simulink model "slave_ctrl"  (Simulink 6.4)
settings: Solver=FixedStepDiscrete  SolverMode=SingleTasking  StartTime=0  StopTime=inf  FixedStep=0.001  RelTol=1e-3
libraries: ecrobot_nxt_lib x9
CloseFcn:
  | rtwprivate ssgencode ModelCloseRequest TestBluetooth
settings Model: Creator=tchikama  LastModifiedBy=tchikama  ProdHWDeviceType=ARM7
settings DataIOCC: SaveOutput=off  SignalLogging=off  SaveTime=off
settings OptimizationCC: InlineParams=on  InlineInvariantSignals=on  RollThreshold=2  StateBitsets=on  DataBitsets=on  UseTempVars=on  InitFltsAndDblsToZero=off  NoFixptDivByZeroProtection=on  EfficientFloat2IntCast=on  OptimizeModelRefInitCode=on  LifeSpan=1
settings DebuggingCC: ConsistencyChecking=warning  SignalInfNanChecking=warning  ReadBeforeWriteMsg=DisableAll  WriteAfterWriteMsg=DisableAll  WriteAfterReadMsg=DisableAll  AlgebraicLoopMsg=error  CheckExecutionContextPreStartOutputMsg=on  CheckExecutionContextRuntimeOutputMsg=on  SolverPrmCheckMsg=none  SingleTaskRateTransMsg=warning  TasksWithSamePriorityMsg=none  IntegerOverflowMsg=error  ParameterPrecisionLossMsg=none  UnconnectedInputMsg=error  UnconnectedOutputMsg=error  UnconnectedLineMsg=error  UniqueDataStoreMsg=error  BusObjectLabelMismatch=error  RootOutportRequireBusObject=error  ModelReferenceIOMsg=warning  ModelReferenceVersionMismatchMessage=warning  ModelReferenceIOMismatchMessage=warning
settings HardwareCC: ProdIntDivRoundTo=Zero  ProdEndianess=LittleEndian  ProdHWDeviceType=ARM7  TargetHWDeviceType=32-bit Generic
settings ModelReferenceCC: ModelReferenceNumInstancesAllowed=Single
settings RTWCC: SystemTargetFile=ert.tlc  GenCodeOnly=on  GenerateMakefile=off  TemplateMakefile=ert_default_tmf  Description=Real-Time Workshop Embedded Coder (no auto configuration)  GenerateReport=on  RTWVerbose=off  ProcessScript=ert_make_rtw_hook  IncludeHyperlinkInReport=on  LaunchReport=on
settings CodeAppCC: ForceParamTrailComments=on  IgnoreCustomStorageClasses=off  SFDataObjDesc=on  PrefixModelToSubsysFcnNames=off  CustomSymbolStrGlobalVar=rt$N$M  CustomSymbolStrType=$N$M  CustomSymbolStrFcn=$N$M$F  CustomSymbolStrMacro=$N$M  InsertBlockDesc=on
settings ERTTargetCC: TargetFcnLib=ansi_tfl_tmw.mat  GenFloatMathFcnCalls=GNU  IncludeMdlTerminateFcn=off  SuppressErrorStatus=on  IncludeERTFirstTime=on  SupportAbsoluteTime=off  SupportNonFinite=off  SupportComplex=off  PurelyIntegerCode=on  InlinedParameterPlacement=NonHierarchical  RootIOFormat=Structure reference  ERTCustomFileTemplate=example_file_process.tlc  InitialValueSource=Model

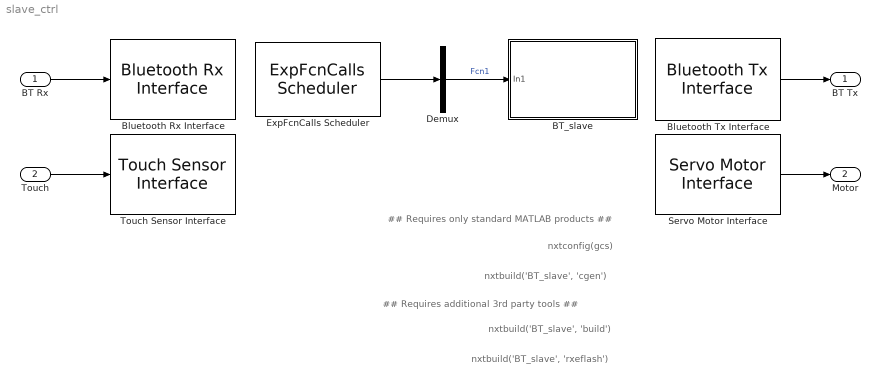
== system slave_ctrl ==
  note: nxtbuild('BT_slave', 'build')
  note: nxtbuild('BT_slave', 'rxeflash')
  note: nxtbuild('BT_slave', 'cgen')
  note: ## Requires only standard MATLAB products ##
  note: ## Requires additional 3rd party tools ##
  note: nxtconfig(gcs)
  BT Rx : Inport  DataType=uint8
  Touch : Inport  Port=2  DataType=uint8
  BT_slave : Subsystem
  Bluetooth Rx Interface : ecrobot_nxt_lib/Bluetooth Rx Interface  SystemSampleTime=-1
  Bluetooth Tx Interface : ecrobot_nxt_lib/Bluetooth Tx Interface  SystemSampleTime=-1
  Demux : Demux  Outputs=1
  ExpFcnCalls Scheduler : ecrobot_nxt_lib/ExpFcnCalls Scheduler  Priority=1  fcname='Fcn1'  fctrigger=[10]  ts=0.001  platform=OSEK  stacksize=[512]  bd_mode=Slave  bd_addr='00', '16', '53', '04', 'F1', 'B3', '00'
  Servo Motor Interface : ecrobot_nxt_lib/Servo Motor Interface  SystemSampleTime=-1  ip=B  mode=Brake
  Touch Sensor Interface : ecrobot_nxt_lib/Touch Sensor Interface  SystemSampleTime=-1  ip=S4
  BT Tx : Outport
  Motor : Outport  Port=2
  wires:
  ExpFcnCalls Scheduler/1 -> Demux/1
  Demux/1 -> BT_slave/1(In1)  "Fcn1"
  BT Rx/1 -> Bluetooth Rx Interface/1
  Bluetooth Tx Interface/1 -> BT Tx/1
  Servo Motor Interface/1 -> Motor/1
  Touch/1 -> Touch Sensor Interface/1

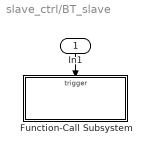
== system slave_ctrl/BT_slave ==
  In1 : Inport  Orientation=down
  Function-Call Subsystem : Subsystem  TreatAsAtomicUnit=on
  wires:
  In1/1 -> Function-Call Subsystem/Trigger

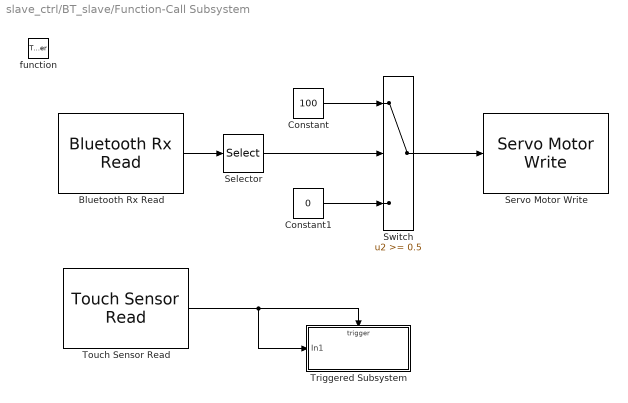
== system slave_ctrl/BT_slave/Function-Call Subsystem ==
  function : TriggerPort  TriggerType=function-call
  Bluetooth Rx Read : ecrobot_nxt_lib/Bluetooth Rx Read
  Constant : Constant  Value=100  OutDataTypeMode=int8  OutDataType=sfix(16)  ConRadixGroup=Use specified scaling  OutScaling=2^0  SampleTime=inf  FramePeriod=inf
  Constant1 : Constant  Value=0  OutDataTypeMode=int8  OutDataType=sfix(16)  ConRadixGroup=Use specified scaling  OutScaling=2^0  SampleTime=inf  FramePeriod=inf
  Selector : Selector  IndexMode=Zero-based  Elements=[0]  InputPortWidth=32
  Servo Motor Write : ecrobot_nxt_lib/Servo Motor Write  SystemSampleTime=-1  ip=B
  Switch : Switch  Threshold=0.5
  Touch Sensor Read : ecrobot_nxt_lib/Touch Sensor Read  SystemSampleTime=-1  ip=S4
  Triggered Subsystem : Subsystem  TreatAsAtomicUnit=on
  wires:
  Bluetooth Rx Read/1 -> Selector/1
  Selector/1 -> Switch/2
  Constant/1 -> Switch/1
  Constant1/1 -> Switch/3
  Switch/1 -> Servo Motor Write/1
  Touch Sensor Read/1 -> Triggered Subsystem/Trigger, Triggered Subsystem/1(In1)

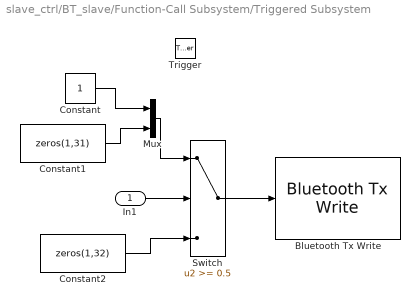
== system slave_ctrl/BT_slave/Function-Call Subsystem/Triggered Subsystem ==
  In1 : Inport
  Trigger : TriggerPort  TriggerType=either
  Bluetooth Tx Write : ecrobot_nxt_lib/Bluetooth Tx Write
  Constant : Constant  Value=1  OutDataTypeMode=uint8  OutDataType=sfix(16)  ConRadixGroup=Use specified scaling  OutScaling=2^0  SampleTime=inf  FramePeriod=inf
  Constant1 : Constant  Value=zeros(1,31)  OutDataTypeMode=uint8  OutDataType=sfix(16)  ConRadixGroup=Use specified scaling  OutScaling=2^0  SampleTime=inf  FramePeriod=inf
  Constant2 : Constant  Value=zeros(1,32)  OutDataTypeMode=uint8  OutDataType=sfix(16)  ConRadixGroup=Use specified scaling  OutScaling=2^0  SampleTime=inf  FramePeriod=inf
  Mux : Mux  Inputs=2
  Switch : Switch  Threshold=0.5
  wires:
  Switch/1 -> Bluetooth Tx Write/1
  In1/1 -> Switch/2
  Constant2/1 -> Switch/3
  Mux/1 -> Switch/1
  Constant/1 -> Mux/1
  Constant1/1 -> Mux/2
